simulink model "IEEE30_case"  (R2024b)
settings: Solver=FixedStepAuto  StartTime=0  StopTime=5  FixedStep=1e-7  RelTol=1e-3
values from neighbouring files (symbols this model uses):
  GFL_DFIG_7_C_bus = 0.08    [IEEE30_case_parameters.m]
  GFL_DFIG_7_D_mutual = 2.500000e+3    (= 2500)    [IEEE30_case_parameters.m]
  GFL_DFIG_7_f0 = 60    [IEEE30_case_parameters.m]
  GFL_DFIG_7_gPLLi = 3200    [IEEE30_case_parameters.m]
  GFL_DFIG_7_gPLLp = 650    [IEEE30_case_parameters.m]
  GFL_DFIG_7_H_WT = 0.4    [IEEE30_case_parameters.m]
  GFL_DFIG_7_Hg = 0.8    [IEEE30_case_parameters.m]
  GFL_DFIG_7_Igq_ref = 0    [IEEE30_case_parameters.m]
  GFL_DFIG_7_Ird_ref = 704.45696    [IEEE30_case_parameters.m]
  GFL_DFIG_7_KI_V = -300000    [IEEE30_case_parameters.m]
  GFL_DFIG_7_KP_V = -1000    [IEEE30_case_parameters.m]
  GFL_DFIG_7_Ksh = 1.254300e+4    (= 12543)    [IEEE30_case_parameters.m]
  GFL_DFIG_7_Lg = 0.000483    [IEEE30_case_parameters.m]
  GFL_DFIG_7_Lm_pu = 4    [IEEE30_case_parameters.m]
  GFL_DFIG_7_N = 100    [IEEE30_case_parameters.m]
  GFL_DFIG_7_p = 2    [IEEE30_case_parameters.m]
  GFL_DFIG_7_Pitch = 0    [IEEE30_case_parameters.m]
  GFL_DFIG_7_R = 44    [IEEE30_case_parameters.m]
  GFL_DFIG_7_Rg = 2.000000e-5    (= 2e-05)    [IEEE30_case_parameters.m]
  GFL_DFIG_7_rho = 1.225    [IEEE30_case_parameters.m]
  GFL_DFIG_7_rPLLi = 4500    [IEEE30_case_parameters.m]
  GFL_DFIG_7_rPLLp = 620    [IEEE30_case_parameters.m]
  GFL_DFIG_7_Rs_pu = 0.011    [IEEE30_case_parameters.m]
  GFL_DFIG_7_Sbase = 2.000000e+6    (= 2000000)    [IEEE30_case_parameters.m]
  GFL_DFIG_7_ugq_ref = 0    [IEEE30_case_parameters.m]
  GFL_DFIG_7_usd_ref = 0    [IEEE30_case_parameters.m]
  GFL_DFIG_7_Vbase = 690    [IEEE30_case_parameters.m]
  GFL_DFIG_7_Vdc_ref = 1200    [IEEE30_case_parameters.m]
  GFL_DFIG_7_wind = 12    [IEEE30_case_parameters.m]
  GFL_DFIG_7_wm_ref = 518.184209    [IEEE30_case_parameters.m]
  SG_D_13_D = 0.01056    [IEEE30_case_parameters.m]
  SG_D_13_EnableSaturation = 0    [IEEE30_case_parameters.m]
  SG_D_13_f0 = 60    [IEEE30_case_parameters.m]
  SG_D_13_H = 7.5    [IEEE30_case_parameters.m]
  SG_D_13_K_A = 20    [IEEE30_case_parameters.m]
  SG_D_13_K_E = 1.000000e+1    (= 10)    [IEEE30_case_parameters.m]
  SG_D_13_K_F = 2.363    [IEEE30_case_parameters.m]
  SG_D_13_K_s = 0.5    [IEEE30_case_parameters.m]
  SG_D_13_R_a = 0.001088    [IEEE30_case_parameters.m]
  SG_D_13_S_A = 1    [IEEE30_case_parameters.m]
  SG_D_13_S_B = 0.103    [IEEE30_case_parameters.m]
  SG_D_13_S_N = 10.659857    [IEEE30_case_parameters.m]
  SG_D_13_SpeedPara = 200    [IEEE30_case_parameters.m]
  SG_D_13_T_0 = 0.370163    [IEEE30_case_parameters.m]
  SG_D_13_T_1 = 0.3    [IEEE30_case_parameters.m]
  SG_D_13_T_2 = 0.05    [IEEE30_case_parameters.m]
  SG_D_13_T_3 = 0.02    [IEEE30_case_parameters.m]
  SG_D_13_T_4 = 0.005    [IEEE30_case_parameters.m]
  SG_D_13_T_A = 0.02    [IEEE30_case_parameters.m]
  SG_D_13_T_dd = 8.000000e+0    (= 8)    [IEEE30_case_parameters.m]
  SG_D_13_T_ddd = 0.04    [IEEE30_case_parameters.m]
  SG_D_13_T_E = 0.314    [IEEE30_case_parameters.m]
  SG_D_13_T_F = 0.35    [IEEE30_case_parameters.m]
  SG_D_13_T_qd = 0.8    [IEEE30_case_parameters.m]
  SG_D_13_T_qdd = 0.02    [IEEE30_case_parameters.m]
  SG_D_13_T_speed = 0.1    [IEEE30_case_parameters.m]
  SG_D_13_T_w = 0.5    [IEEE30_case_parameters.m]
  SG_D_13_V_ref = 1.696619    [IEEE30_case_parameters.m]
  SG_D_13_w_ref = 376.991118    [IEEE30_case_parameters.m]
  SG_D_13_x_d = 1.9    [IEEE30_case_parameters.m]
  SG_D_13_x_dd = 0.302    [IEEE30_case_parameters.m]
  SG_D_13_x_ddd = 0.204    [IEEE30_case_parameters.m]
  SG_D_13_x_l = 0.05    [IEEE30_case_parameters.m]
  SG_D_13_x_q = 1.3    [IEEE30_case_parameters.m]
  SG_D_13_x_qd = 0.5    [IEEE30_case_parameters.m]
  SG_D_13_x_qdd = 0.3    [IEEE30_case_parameters.m]
  SG_D_1_D = 0.01056    [IEEE30_case_parameters.m]
  SG_D_1_EnableSaturation = 0    [IEEE30_case_parameters.m]
  SG_D_1_f0 = 60    [IEEE30_case_parameters.m]
  SG_D_1_H = 7.5    [IEEE30_case_parameters.m]
  SG_D_1_K_A = 20    [IEEE30_case_parameters.m]
  SG_D_1_K_E = 1.000000e+1    (= 10)    [IEEE30_case_parameters.m]
  SG_D_1_K_F = 2.363    [IEEE30_case_parameters.m]
  SG_D_1_K_s = 0.5    [IEEE30_case_parameters.m]
  SG_D_1_R_a = 0.001088    [IEEE30_case_parameters.m]
  SG_D_1_S_A = 1    [IEEE30_case_parameters.m]
  SG_D_1_S_B = 0.103    [IEEE30_case_parameters.m]
  SG_D_1_S_N = 10.659857    [IEEE30_case_parameters.m]
  SG_D_1_SpeedPara = 200    [IEEE30_case_parameters.m]
  SG_D_1_T_0 = 0.259812    [IEEE30_case_parameters.m]
  SG_D_1_T_1 = 0.3    [IEEE30_case_parameters.m]
  SG_D_1_T_2 = 0.05    [IEEE30_case_parameters.m]
  SG_D_1_T_3 = 0.02    [IEEE30_case_parameters.m]
  SG_D_1_T_4 = 0.005    [IEEE30_case_parameters.m]
  SG_D_1_T_A = 0.02    [IEEE30_case_parameters.m]
  SG_D_1_T_dd = 8.000000e+0    (= 8)    [IEEE30_case_parameters.m]
  SG_D_1_T_ddd = 0.04    [IEEE30_case_parameters.m]
  SG_D_1_T_E = 0.314    [IEEE30_case_parameters.m]
  SG_D_1_T_F = 0.35    [IEEE30_case_parameters.m]
  SG_D_1_T_qd = 0.8    [IEEE30_case_parameters.m]
  SG_D_1_T_qdd = 0.02    [IEEE30_case_parameters.m]
  SG_D_1_T_speed = 0.1    [IEEE30_case_parameters.m]
  SG_D_1_T_w = 0.5    [IEEE30_case_parameters.m]
  SG_D_1_V_ref = 1.544107    [IEEE30_case_parameters.m]
  SG_D_1_w_ref = 376.991118    [IEEE30_case_parameters.m]
  SG_D_1_x_d = 1.9    [IEEE30_case_parameters.m]
  SG_D_1_x_dd = 0.302    [IEEE30_case_parameters.m]
  SG_D_1_x_ddd = 0.204    [IEEE30_case_parameters.m]
  SG_D_1_x_l = 0.05    [IEEE30_case_parameters.m]
  SG_D_1_x_q = 1.3    [IEEE30_case_parameters.m]
  SG_D_1_x_qd = 0.5    [IEEE30_case_parameters.m]
  SG_D_1_x_qdd = 0.3    [IEEE30_case_parameters.m]
  SG_D_22_D = 0.01056    [IEEE30_case_parameters.m]
  SG_D_22_EnableSaturation = 0    [IEEE30_case_parameters.m]
  SG_D_22_f0 = 60    [IEEE30_case_parameters.m]
  SG_D_22_H = 7.5    [IEEE30_case_parameters.m]
  SG_D_22_K_A = 20    [IEEE30_case_parameters.m]
  SG_D_22_K_E = 1.000000e+1    (= 10)    [IEEE30_case_parameters.m]
  SG_D_22_K_F = 2.363    [IEEE30_case_parameters.m]
  SG_D_22_K_s = 0.5    [IEEE30_case_parameters.m]
  SG_D_22_R_a = 0.001088    [IEEE30_case_parameters.m]
  SG_D_22_S_A = 1    [IEEE30_case_parameters.m]
  SG_D_22_S_B = 0.103    [IEEE30_case_parameters.m]
  SG_D_22_S_N = 10.659857    [IEEE30_case_parameters.m]
  SG_D_22_SpeedPara = 200    [IEEE30_case_parameters.m]
  SG_D_22_T_0 = 0.216121    [IEEE30_case_parameters.m]
  SG_D_22_T_1 = 0.3    [IEEE30_case_parameters.m]
  SG_D_22_T_2 = 0.05    [IEEE30_case_parameters.m]
  SG_D_22_T_3 = 0.02    [IEEE30_case_parameters.m]
  SG_D_22_T_4 = 0.005    [IEEE30_case_parameters.m]
  ... (+126 more)
(part 13 of 27)

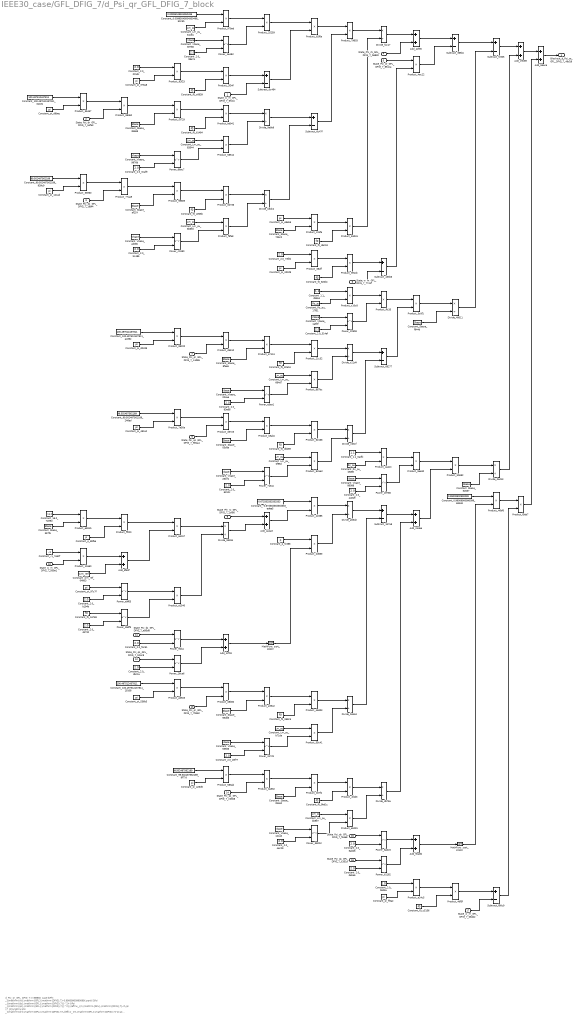
== system IEEE30_case/GFL_DFIG_7/d_Psi_qr_GFL_DFIG_7_block ==
  note: d_Psi_qr_GFL_DFIG_7 in IEEE30_case
      | $\Phi _{\mathrm{rb},\mathrm{GFL},\mathrm{DFIG},7}-0.99009900990099\,\sqrt{{\Psi _{\mathrm{ds},\mathrm{GFL},\mathrm{DFIG},7}}^2+{\Psi _{\mathrm{qs},\mathrm{GFL},\mathrm{DFIG},7}}^2}\,\left(w_{m,\mathrm{GFL},\mathrm{DFIG},7}-2\,\pi \,f_{0}\right)+\Psi _{\mathrm{dr},\mathrm{GFL},\mathrm{DFIG},7}\,\left(w_{m,\mathrm{GFL},\mathrm{DFIG},7}-2\,\pi \,f_{0}\right)-\frac{1.1\,\mathrm{Rs}_{\mathrm{pu}}\,{\mathrm{Vbase}}^2\,\left(\frac{100.497512437811\,\pi \,\Psi _{\mathrm{qr},\mathrm{GFL},\mathrm{DFIG},7}\,\mathrm{Sbase}\,f_{0}}{\mathrm{Lm}_{\mathrm{pu}}\,{\mathrm{Vbase}}^2}-\frac{99.502487562189\,\pi \,\Psi _{\mathrm{qs},\mathrm{GFL},\mathrm{DFIG},7}\,\mathrm{Sbase}\,f_{0}}{\mathrm{Lm}_{\mathrm{pu}}\,{\mathrm{Vbase}}^2}\right)}{\mathrm{Sbase}}-\frac{1.1\,\mathrm{Rs}_{\mathrm{pu}}\,{\mathrm{Vbase}}^2\,\left(\frac{0.673333333333333\,\Phi _{\mathrm{rc},\mathrm{GFL},\mathrm{DFIG},7}-\frac{10.773333333333328\,\mathrm{Sbase}\,p\,\left(w_{m,\mathrm{GFL},\mathrm{DFIG},7}-\mathrm{wm}_{\mathrm{ref}}\right)}{{f_{0}}^2\,\pi ^2}}{p\,\sqrt{{\Psi _{\mathrm{ds},\mathrm{GFL},\mathrm{DFIG},7}}^2+{\Psi _{\mathrm{qs},\mathrm{GFL},\mathrm{DFIG},7}}^2}}+\frac{100.497512437811\,\pi \,\Psi _{\mathrm{qr},\mathrm{GFL},\mathrm{DFIG},7}\,\mathrm{Sbase}\,f_{0}}{\mathrm{Lm}_{\mathrm{pu}}\,{\mathrm{Vbase}}^2}-\frac{99.502487562189\,\pi \,\Psi _{\mathrm{qs},\mathrm{GFL},\mathrm{DFIG},7}\,\mathrm{Sbase}\,f_{0}}{\mathrm{Lm}_{\mathrm{pu}}\,{\mathrm{Vbase}}^2}\right)}{\mathrm{Sbase}}-\frac{0.00995049504950496\,\mathrm{Lm}_{\mathrm{pu}}\,{\mathrm{Vbase}}^2\,\left(\frac{100.497512437811\,\pi \,\Psi _{\mathrm{dr},\mathrm{GFL},\mathrm{DFIG},7}\,\mathrm{Sbase}\,f_{0}}{\mathrm{Lm}_{\mathrm{pu}}\,{\mathrm{Vbase}}^2}-\frac{99.502487562189\,\pi \,\Psi _{\mathrm{ds},\mathrm{GFL},\mathrm{DFIG},7}\,\mathrm{Sbase}\,f_{0}}{\mathrm{Lm}_{\mathrm{pu}}\,{\mathrm{Vbase}}^2}\right)\,\left(w_{m,\mathrm{GFL},\mathrm{DFIG},7}-2\,\pi \,f_{0}\right)}{\mathrm{Sbase}\,f_{0}\,\pi }$
      | Automatically generated on 2025-11-01 18:33:02 .
  State_w_m_GFL_DFIG_7_5fc1b : Inport
  State_Psi_dr_GFL_DFIG_7_54fa3 : Inport  Port=2
  State_Psi_ds_GFL_DFIG_7_18bf4 : Inport  Port=3
  State_Phi_rb_GFL_DFIG_7_b6830 : Inport  Port=4
  State_Psi_dr_GFL_DFIG_7_851ca : Inport  Port=5
  State_w_m_GFL_DFIG_7_7741f : Inport  Port=6
  State_Psi_qr_GFL_DFIG_7_c4d86 : Inport  Port=7
  State_Psi_qs_GFL_DFIG_7_981a4 : Inport  Port=8
  State_Phi_rc_GFL_DFIG_7_1cf80 : Inport  Port=9
  State_w_m_GFL_DFIG_7_509a1 : Inport  Port=10
  State_Psi_ds_GFL_DFIG_7_e95d8 : Inport  Port=11
  State_Psi_qs_GFL_DFIG_7_b24c8 : Inport  Port=12
  State_Psi_qr_GFL_DFIG_7_7bb62 : Inport  Port=13
  State_Psi_qs_GFL_DFIG_7_c0308 : Inport  Port=14
  State_Psi_ds_GFL_DFIG_7_fa3e8 : Inport  Port=15
  State_Psi_qs_GFL_DFIG_7_c351a : Inport  Port=16
  State_w_m_GFL_DFIG_7_084b2 : Inport  Port=17
  Add_1cf03 : Sum
  Add_24dee : Sum
  Add_42f35 : Sum
  Add_4a1a3 : Sum
  Add_55ace : Sum
  Add_8fe3f : Sum
  Add_9ca6b : Sum
  Add_c9c89 : Sum
  Constant_-0.673333333333333_edee5 : Constant  Value=-0.673333333333333
  Constant_-1_7e52f : Constant  Value=-1
  Constant_0.00995049504950496_52c5b : Constant  Value=0.00995049504950496
  Constant_0.99009900990099_a5b48 : Constant  Value=0.99009900990099
  Constant_1.1_0adfc : Constant  Value=1.1
  Constant_1.1_db8a1 : Constant  Value=1.1
  Constant_100.497512437811_19108 : Constant  Value=100.497512437811
  Constant_100.497512437811_34181 : Constant  Value=100.497512437811
  Constant_100.497512437811_a4362 : Constant  Value=100.497512437811
  Constant_16.0_72e9d : Constant  Value=16.0
  Constant_2.0_001dc : Constant  Value=2.0
  Constant_2.0_0caf9 : Constant  Value=2.0
  Constant_2.0_28f77 : Constant  Value=2.0
  Constant_2.0_314ef : Constant  Value=2.0
  Constant_2.0_44819 : Constant  Value=2.0
  Constant_2.0_4b732 : Constant  Value=2.0
  Constant_2.0_4ec29 : Constant  Value=2.0
  Constant_2.0_5abb6 : Constant  Value=2.0
  Constant_2.0_6312c : Constant  Value=2.0
  Constant_2.0_73f2b : Constant  Value=2.0
  Constant_2.0_83e68 : Constant  Value=2.0
  Constant_2.0_99e74 : Constant  Value=2.0
  Constant_2.0_b194b : Constant  Value=2.0
  Constant_2.0_b505a : Constant  Value=2.0
  Constant_2.0_bc485 : Constant  Value=2.0
  Constant_2.0_dbc1a : Constant  Value=2.0
  Constant_2.0_deba6 : Constant  Value=2.0
  Constant_2.0_f4c51 : Constant  Value=2.0
  Constant_99.502487562189_246ed : Constant  Value=99.502487562189
  Constant_99.502487562189_939c9 : Constant  Value=99.502487562189
  Constant_99.502487562189_9f77d : Constant  Value=99.502487562189
  Constant_Lm_pu_0f95d : Constant  Value=Lm_pu
  Constant_Lm_pu_664d7 : Constant  Value=Lm_pu
  Constant_Lm_pu_83544 : Constant  Value=Lm_pu
  Constant_Lm_pu_8b6ed : Constant  Value=Lm_pu
  Constant_Lm_pu_b71da : Constant  Value=Lm_pu
  Constant_Lm_pu_bb9e7 : Constant  Value=Lm_pu
  Constant_Lm_pu_e4c81 : Constant  Value=Lm_pu
  Constant_Rs_pu_17f51 : Constant  Value=Rs_pu
  Constant_Rs_pu_b58f8 : Constant  Value=Rs_pu
  Constant_Sbase_05cea : Constant  Value=Sbase
  Constant_Sbase_0ba52 : Constant  Value=Sbase
  Constant_Sbase_357fe : Constant  Value=Sbase
  Constant_Sbase_3b669 : Constant  Value=Sbase
  Constant_Sbase_52637 : Constant  Value=Sbase
  Constant_Sbase_705c0 : Constant  Value=Sbase
  Constant_Sbase_8fae6 : Constant  Value=Sbase
  Constant_Sbase_9ed05 : Constant  Value=Sbase
  Constant_Sbase_af214 : Constant  Value=Sbase
  Constant_Sbase_f944d : Constant  Value=Sbase
  Constant_Vbase_12ca0 : Constant  Value=Vbase
  Constant_Vbase_1ae0f : Constant  Value=Vbase
  Constant_Vbase_204ae : Constant  Value=Vbase
  Constant_Vbase_25b72 : Constant  Value=Vbase
  Constant_Vbase_3e766 : Constant  Value=Vbase
  Constant_Vbase_55566 : Constant  Value=Vbase
  Constant_Vbase_860d8 : Constant  Value=Vbase
  Constant_Vbase_9976d : Constant  Value=Vbase
  Constant_Vbase_ad08c : Constant  Value=Vbase
  Constant_f0_068c5 : Constant  Value=f0
  Constant_f0_16769 : Constant  Value=f0
  Constant_f0_32a04 : Constant  Value=f0
  Constant_f0_4e06b : Constant  Value=f0
  Constant_f0_820bc : Constant  Value=f0
  Constant_f0_9bd1c : Constant  Value=f0
  Constant_f0_b1484 : Constant  Value=f0
  Constant_f0_c5156 : Constant  Value=f0
  Constant_f0_c6639 : Constant  Value=f0
  Constant_f0_d6c18 : Constant  Value=f0
  Constant_f0_dbb69 : Constant  Value=f0
  Constant_p_6bf5e : Constant  Value=p
  Constant_p_fc388 : Constant  Value=p
  Constant_pi_12cad : Constant  Value=pi
  Constant_pi_2d2d9 : Constant  Value=pi
  Constant_pi_37ea8 : Constant  Value=pi
  Constant_pi_426d6 : Constant  Value=pi
  Constant_pi_491a2 : Constant  Value=pi
  Constant_pi_536b5 : Constant  Value=pi
  Constant_pi_97c7f : Constant  Value=pi
  Constant_pi_d0c89 : Constant  Value=pi
  Constant_pi_d9bec : Constant  Value=pi
  Constant_pi_e9eb6 : Constant  Value=pi
  Constant_pi_ff3a2 : Constant  Value=pi
  Constant_wm_ref_04b03 : Constant  Value=wm_ref
  Divide_0ad13 : Product  Inputs=*/
  Divide_48011 : Product  Inputs=*/
  Divide_93334 : Product  Inputs=*/
  Divide_9abb9 : Product  Inputs=*/
  Divide_a55d2 : Product  Inputs=*/
  Divide_b34a3 : Product  Inputs=*/
  Divide_b3dc2 : Product  Inputs=*/
  Divide_c03cf : Product  Inputs=*/
  Divide_c21d4 : Product  Inputs=*/
  Divide_db75a : Product  Inputs=*/
  Divide_f4c17 : Product  Inputs=*/
  MathFunc_sqrt_20207 : Sqrt
  MathFunc_sqrt_c0122 : Sqrt
  Power_1e48d : Math  Operator=pow
  Power_225b9 : Math  Operator=pow
  Power_26ca6 : Math  Operator=pow
  Power_2e786 : Math  Operator=pow
  Power_317d1 : Math  Operator=pow
  Power_3602d : Math  Operator=pow
  Power_36df3 : Math  Operator=pow
  Power_66ac7 : Math  Operator=pow
  Power_6a0c6 : Math  Operator=pow
  Power_7161c : Math  Operator=pow
  Power_a9f63 : Math  Operator=pow
  Power_b1182 : Math  Operator=pow
  Power_c1590 : Math  Operator=pow
  Power_e3aa1 : Math  Operator=pow
  Power_ffbb4 : Math  Operator=pow
  Product_0d736 : Product
  Product_{11660,25259,35457,42385,58512,62168,79603,99220} (8 alike) : Product
  Product_21c32 : Product
  Product_2d65e : Product
  Product_2f34f : Product
  Product_384ff : Product
  Product_391dc : Product
  Product_3c0f1 : Product
  Product_3ee60 : Product
  Product_46bf0 : Product
  Product_46dd3 : Product
  Product_4a42c : Product
  Product_4ac22 : Product
  Product_4df3f : Product
  Product_4f4d3 : Product
  Product_53dc6 : Product
  Product_55c41 : Product
  Product_583ab : Product
  Product_641b7 : Product
  Product_774a9 : Product
  Product_7a50a : Product
  Product_887bc : Product
  Product_92f23 : Product
  Product_979ad : Product
  Product_98de2 : Product
  Product_9ae30 : Product
  Product_9c5ed : Product
  Product_9e8ee : Product
  Product_a0503 : Product
  Product_a24c5 : Product
  Product_a2540 : Product
  Product_a3542 : Product
  Product_a7124 : Product
  Product_b07f2 : Product
  Product_b2f6a : Product
  Product_ba532 : Product
  Product_bb592 : Product
  Product_bd941 : Product
  Product_beabc : Product
  Product_c04fe : Product
  Product_c10c8 : Product
  Product_d5510 : Product
  Product_d5723 : Product
  Product_d8b60 : Product
  Product_e5291 : Product
  Product_e831b : Product
  Product_f3729 : Product
  Product_f5eb7 : Product
  Product_f9fa8 : Product
  Product_ff020 : Product
  Product_ffc35 : Product
  Subtract_0c464 : Sum  Inputs=+-
  Subtract_1b7a8 : Sum  Inputs=+-
  Subtract_365bc : Sum  Inputs=+-
  Subtract_433b6 : Sum  Inputs=+-
  Subtract_66277 : Sum  Inputs=+-
  Subtract_6c47f : Sum  Inputs=+-
  Subtract_f80c9 : Sum  Inputs=+-
  Subtract_fc605 : Sum  Inputs=+-
  Blockout_d_Psi_qr_GFL_DFIG_7_49d19 : Outport
  wires:
  Constant_2.0_5abb6/1 -> Power_6a0c6/2
  Constant_1.1_db8a1/1 -> Product_c10c8/1
  Constant_Vbase_55566/1 -> Power_317d1/1
  State_Psi_qs_GFL_DFIG_7_b24c8/1 -> Power_26ca6/1
  Add_55ace/1 -> Blockout_d_Psi_qr_GFL_DFIG_7_49d19/1
  Constant_Lm_pu_bb9e7/1 -> Product_e5291/1
  Add_42f35/1 -> Subtract_365bc/1
  State_Psi_qr_GFL_DFIG_7_c4d86/1 -> Product_d5510/2
  Power_b1182/1 -> Add_9ca6b/2
  Power_3602d/1 -> Product_e5291/2
  Constant_Vbase_204ae/1 -> Power_e3aa1/1
  Subtract_f80c9/1 -> Product_f5eb7/2
  Product_3ee60/1 -> Product_774a9/1
  Product_42385/1 -> Divide_a55d2/1
  Product_4df3f/1 -> Subtract_f80c9/1
  Product_f5eb7/1 -> Add_55ace/2
  Constant_Lm_pu_b71da/1 -> Product_55c41/1
  Product_92f23/1 -> Product_2f34f/1
  MathFunc_sqrt_c0122/1 -> Product_46bf0/2
  Add_1cf03/1 -> MathFunc_sqrt_20207/1
  State_w_m_GFL_DFIG_7_084b2/1 -> Subtract_f80c9/2
  Divide_a55d2/1 -> Subtract_1b7a8/1
  Product_46bf0/1 -> Product_f5eb7/1
  Constant_2.0_dbc1a/1 -> Power_26ca6/2
  Product_11660/1 -> Add_8fe3f/1
  Add_24dee/1 -> Product_bb592/2
  Constant_Vbase_12ca0/1 -> Power_3602d/1
  Constant_0.99009900990099_a5b48/1 -> Product_46bf0/1
  Constant_f0_c5156/1 -> Product_4df3f/2
  Add_9ca6b/1 -> MathFunc_sqrt_c0122/1
  Constant_p_fc388/1 -> Product_2d65e/1
  Constant_pi_ff3a2/1 -> Product_a24c5/2
  Constant_Sbase_0ba52/1 -> Product_b07f2/2
  Product_a24c5/1 -> Product_4df3f/1
  Product_9ae30/1 -> Product_bb592/1
  Constant_2.0_b505a/1 -> Product_a24c5/1
  Power_317d1/1 -> Product_55c41/2
  Constant_pi_426d6/1 -> Product_583ab/2
  Divide_0ad13/1 -> Add_c9c89/2
  State_Psi_qs_GFL_DFIG_7_c351a/1 -> Power_b1182/1
  Product_ba532/1 -> Product_b07f2/1
  Constant_100.497512437811_19108/1 -> Product_a0503/1
  State_Phi_rb_GFL_DFIG_7_b6830/1 -> Add_42f35/2
  Constant_2.0_deba6/1 -> Power_b1182/2
  Constant_2.0_0caf9/1 -> Power_66ac7/2
  Constant_Vbase_1ae0f/1 -> Power_225b9/1
  State_Psi_qs_GFL_DFIG_7_c0308/1 -> Product_ba532/2
  Divide_db75a/1 -> Add_24dee/2
  Product_53dc6/1 -> Divide_f4c17/2
  Product_21c32/1 -> Divide_c21d4/1
  Constant_99.502487562189_9f77d/1 -> Product_583ab/1
  Constant_100.497512437811_34181/1 -> Product_35457/1
  Constant_f0_9bd1c/1 -> Product_4f4d3/2
  Constant_pi_d0c89/1 -> Product_99220/2
  Power_6a0c6/1 -> Add_9ca6b/1
  Product_bb592/1 -> Divide_0ad13/1
  Product_bd941/1 -> Divide_9abb9/1
  Product_583ab/1 -> Product_ba532/1
  Product_9c5ed/1 -> Divide_c03cf/2
  Product_98de2/1 -> Product_f3729/1
  State_Psi_ds_GFL_DFIG_7_fa3e8/1 -> Power_6a0c6/1
  Product_b07f2/1 -> Product_4f4d3/1
  Add_8fe3f/1 -> Product_641b7/2
  Constant_f0_d6c18/1 -> Product_53dc6/2
  Constant_f0_068c5/1 -> Product_46dd3/2
  Constant_Sbase_52637/1 -> Divide_0ad13/2
  Add_c9c89/1 -> Add_55ace/1
  Product_46dd3/1 -> Divide_b34a3/1
  Constant_2.0_314ef/1 -> Power_225b9/2
  Product_e5291/1 -> Divide_db75a/2
  Constant_2.0_4ec29/1 -> Power_3602d/2
  Product_4f4d3/1 -> Divide_db75a/1
  Product_4ac22/1 -> Subtract_365bc/2
  Constant_pi_536b5/1 -> Product_a0503/2
  Subtract_1b7a8/1 -> Add_24dee/1
  Constant_pi_2d2d9/1 -> Product_384ff/2
  Product_391dc/1 -> Subtract_433b6/1
  Constant_f0_820bc/1 -> Product_391dc/2
  Divide_b34a3/1 -> Subtract_1b7a8/2
  Product_55c41/1 -> Divide_b34a3/2
  Constant_2.0_28f77/1 -> Power_317d1/2
  Product_a3542/1 -> Product_46dd3/1
  Constant_2.0_f4c51/1 -> Power_ffbb4/2
  Constant_Sbase_9ed05/1 -> Product_a3542/2
  Power_ffbb4/1 -> Add_1cf03/1
  Product_d8b60/1 -> Product_a3542/1
  State_Psi_qr_GFL_DFIG_7_7bb62/1 -> Product_d8b60/2
  Product_a0503/1 -> Product_d8b60/1
  Product_2d65e/1 -> Divide_a55d2/2
  MathFunc_sqrt_20207/1 -> Product_2d65e/2
  Constant_Vbase_3e766/1 -> Power_1e48d/1
  Power_26ca6/1 -> Add_1cf03/2
  Product_f9fa8/1 -> Divide_b3dc2/2
  State_Psi_ds_GFL_DFIG_7_e95d8/1 -> Power_ffbb4/1
  Constant_pi_e9eb6/1 -> Product_c04fe/1
  Constant_2.0_44819/1 -> Power_2e786/2
  Add_4a1a3/1 -> Product_42385/2
  Power_7161c/1 -> Product_9c5ed/2
  Divide_93334/1 -> Add_4a1a3/2
  Product_a2540/1 -> Divide_93334/2
  Constant_Sbase_05cea/1 -> Product_beabc/2
  Subtract_fc605/1 -> Add_c9c89/1
  Power_36df3/1 -> Product_a2540/2
  Constant_2.0_4b732/1 -> Power_36df3/2
  Constant_p_6bf5e/1 -> Product_ff020/2
  Constant_f0_16769/1 -> Power_36df3/1
  Power_a9f63/1 -> Product_a2540/1
  Constant_2.0_b194b/1 -> Power_a9f63/2
  Constant_Lm_pu_0f95d/1 -> Product_9c5ed/1
  Power_2e786/1 -> Product_9ae30/2
  Constant_pi_97c7f/1 -> Power_a9f63/1
  Product_641b7/1 -> Divide_93334/1
  Constant_2.0_6312c/1 -> Power_7161c/2
  Constant_wm_ref_04b03/1 -> Add_8fe3f/2
  State_w_m_GFL_DFIG_7_509a1/1 -> Product_11660/2
  Constant_-1_7e52f/1 -> Product_11660/1
  Product_ff020/1 -> Product_641b7/1
  Product_e831b/1 -> Product_ff020/1
  Product_58512/1 -> Divide_9abb9/2
  Constant_Sbase_357fe/1 -> Product_e831b/2
  Constant_16.0_72e9d/1 -> Product_e831b/1
  State_Phi_rc_GFL_DFIG_7_1cf80/1 -> Add_4a1a3/1
  Constant_-0.673333333333333_edee5/1 -> Product_42385/1
  Constant_Vbase_860d8/1 -> Power_2e786/1
  Product_4a42c/1 -> Product_9ae30/1
  Product_2f34f/1 -> Subtract_0c464/1
  Constant_Rs_pu_b58f8/1 -> Product_4a42c/2
  Constant_1.1_0adfc/1 -> Product_4a42c/1
  Divide_48011/1 -> Subtract_fc605/2
  Subtract_6c47f/1 -> Product_79603/2
  Constant_Sbase_f944d/1 -> Divide_48011/2
  Product_3c0f1/1 -> Divide_48011/1
  Subtract_66277/1 -> Product_3c0f1/2
  Constant_Lm_pu_8b6ed/1 -> Product_f9fa8/1
  Product_62168/1 -> Divide_c03cf/1
  Divide_c03cf/1 -> Subtract_66277/2
  Constant_Vbase_25b72/1 -> Power_7161c/1
  Constant_f0_dbb69/1 -> Product_62168/2
  Product_beabc/1 -> Product_62168/1
  Product_d5723/1 -> Product_beabc/1
  State_Psi_qs_GFL_DFIG_7_981a4/1 -> Product_d5723/2
  Product_7a50a/1 -> Product_d5723/1
  Product_f3729/1 -> Product_bd941/1
  Constant_pi_491a2/1 -> Product_7a50a/2
  Constant_99.502487562189_246ed/1 -> Product_7a50a/1
  Divide_c21d4/1 -> Subtract_66277/1
  Product_887bc/1 -> Divide_c21d4/2
  Power_e3aa1/1 -> Product_887bc/2
  Constant_2.0_83e68/1 -> Power_e3aa1/2
  Constant_Lm_pu_664d7/1 -> Product_887bc/1
  Constant_f0_32a04/1 -> Product_21c32/2
  Product_a7124/1 -> Product_21c32/1
  Product_d5510/1 -> Product_a7124/1
  Constant_Sbase_8fae6/1 -> Product_a7124/2
  Product_99220/1 -> Product_d5510/1
  Subtract_433b6/1 -> Product_4ac22/2
  Constant_f0_c6639/1 -> Product_2f34f/2
  Constant_100.497512437811_a4362/1 -> Product_99220/1
  Product_ffc35/1 -> Product_3c0f1/1
  Power_225b9/1 -> Product_ffc35/2
  Constant_2.0_bc485/1 -> Power_c1590/2
  Product_c10c8/1 -> Product_ffc35/1
  Constant_Rs_pu_17f51/1 -> Product_c10c8/2
  Subtract_365bc/1 -> Subtract_fc605/1
  State_w_m_GFL_DFIG_7_7741f/1 -> Subtract_433b6/2
  State_Psi_ds_GFL_DFIG_7_18bf4/1 -> Product_774a9/2
  Product_384ff/1 -> Product_391dc/1
  Constant_2.0_73f2b/1 -> Product_384ff/1
  State_Psi_dr_GFL_DFIG_7_851ca/1 -> Product_4ac22/1
  Divide_f4c17/1 -> Add_42f35/1
  Product_c04fe/1 -> Product_53dc6/1
  Constant_Sbase_705c0/1 -> Product_c04fe/2
  Product_79603/1 -> Divide_f4c17/1
  Divide_b3dc2/1 -> Subtract_6c47f/2
  Power_1e48d/1 -> Product_25259/2
  Power_c1590/1 -> Product_f9fa8/2
  Constant_Vbase_ad08c/1 -> Power_c1590/1
  Product_0d736/1 -> Divide_b3dc2/1
  Constant_f0_4e06b/1 -> Product_0d736/2
  Product_9e8ee/1 -> Product_0d736/1
  Constant_Sbase_af214/1 -> Product_9e8ee/2
  Product_774a9/1 -> Product_9e8ee/1
  Constant_pi_12cad/1 -> Product_3ee60/2
  Constant_99.502487562189_939c9/1 -> Product_3ee60/1
  Divide_9abb9/1 -> Subtract_6c47f/1
  Power_66ac7/1 -> Product_58512/2
  Constant_Vbase_9976d/1 -> Power_66ac7/1
  Constant_Lm_pu_83544/1 -> Product_58512/1
  Constant_f0_b1484/1 -> Product_bd941/2
  Constant_Sbase_3b669/1 -> Product_f3729/2
  State_Psi_dr_GFL_DFIG_7_54fa3/1 -> Product_98de2/2
  Product_35457/1 -> Product_98de2/1
  Constant_pi_d9bec/1 -> Product_35457/2
  Product_b2f6a/1 -> Product_79603/1
  Subtract_0c464/1 -> Product_b2f6a/2
  State_w_m_GFL_DFIG_7_5fc1b/1 -> Subtract_0c464/2
  Constant_pi_37ea8/1 -> Product_92f23/2
  Constant_2.0_001dc/1 -> Product_92f23/1
  Product_25259/1 -> Product_b2f6a/1
  Constant_2.0_99e74/1 -> Power_1e48d/2
  Product_979ad/1 -> Product_25259/1
  Constant_Lm_pu_e4c81/1 -> Product_979ad/2
  Constant_0.00995049504950496_52c5b/1 -> Product_979ad/1

== system IEEE30_case/GFL_DFIG_7/d_Psi_qs_GFL_DFIG_7_block ==
  note: d_Psi_qs_GFL_DFIG_7 in IEEE30_case
      | $\frac{\mathrm{Rs}_{\mathrm{pu}}\,{\mathrm{Vbase}}^2\,\left(\frac{99.502487562189\,\pi \,\Psi _{\mathrm{qr},\mathrm{GFL},\mathrm{DFIG},7}\,\mathrm{Sbase}\,f_{0}}{\mathrm{Lm}_{\mathrm{pu}}\,{\mathrm{Vbase}}^2}-\frac{100.497512437811\,\pi \,\Psi _{\mathrm{qs},\mathrm{GFL},\mathrm{DFIG},7}\,\mathrm{Sbase}\,f_{0}}{\mathrm{Lm}_{\mathrm{pu}}\,{\mathrm{Vbase}}^2}\right)}{\mathrm{Sbase}}-2\,\pi \,\Psi _{\mathrm{ds},\mathrm{GFL},\mathrm{DFIG},7}\,f_{0}-\mathrm{Vbase}\,\left(v_{q,\mathrm{GFL},\mathrm{DFIG},7}\,\cos\left(\theta _{\mathrm{pllr},\mathrm{GFL},\mathrm{DFIG},7}\right)+v_{d,\mathrm{GFL},\mathrm{DFIG},7}\,\sin\left(\theta _{\mathrm{pllr},\mathrm{GFL},\mathrm{DFIG},7}\right)\right)$
      | Automatically generated on 2025-11-01 18:32:35 .
  State_Psi_ds_GFL_DFIG_7_90de9 : Inport
  State_Psi_qr_GFL_DFIG_7_e0b4f : Inport  Port=2
  State_Psi_qs_GFL_DFIG_7_b8433 : Inport  Port=3
  Input_v_d_GFL_DFIG_7_b1351 : Inport  Port=4
  State_theta_pllr_GFL_DFIG_7_5db89 : Inport  Port=5
  Input_v_q_GFL_DFIG_7_1b265 : Inport  Port=6
  State_theta_pllr_GFL_DFIG_7_ab88b : Inport  Port=7
  Add_05679 : Sum
  Add_d712b : Sum
  Constant_-1_14e2d : Constant  Value=-1
  Constant_-2.0_05158 : Constant  Value=-2.0
  Constant_-99.502487562189_0af13 : Constant  Value=-99.502487562189
  Constant_100.497512437811_b4471 : Constant  Value=100.497512437811
  Constant_2.0_05449 : Constant  Value=2.0
  Constant_2.0_29645 : Constant  Value=2.0
  Constant_2.0_2f381 : Constant  Value=2.0
  Constant_Lm_pu_31d4a : Constant  Value=Lm_pu
  Constant_Lm_pu_97a11 : Constant  Value=Lm_pu
  Constant_Rs_pu_415ee : Constant  Value=Rs_pu
  Constant_Sbase_92d1d : Constant  Value=Sbase
  Constant_Sbase_9cdbc : Constant  Value=Sbase
  Constant_Sbase_c8db8 : Constant  Value=Sbase
  Constant_Vbase_72de1 : Constant  Value=Vbase
  Constant_Vbase_7e994 : Constant  Value=Vbase
  Constant_Vbase_8fefb : Constant  Value=Vbase
  Constant_Vbase_9231f : Constant  Value=Vbase
  Constant_f0_4d31c : Constant  Value=f0
  Constant_f0_be9d9 : Constant  Value=f0
  Constant_f0_e5f2c : Constant  Value=f0
  Constant_pi_34fb3 : Constant  Value=pi
  Constant_pi_6d70d : Constant  Value=pi
  Constant_pi_ac4ca : Constant  Value=pi
  Divide_00334 : Product  Inputs=*/
  Divide_87c86 : Product  Inputs=*/
  Divide_d6566 : Product  Inputs=*/
  MathFunc_cos_a232e : Trigonometry  Operator=cos
  MathFunc_sin_5425e : Trigonometry
  Power_2ce9c : Math  Operator=pow
  Power_417a6 : Math  Operator=pow
  Power_b6549 : Math  Operator=pow
  Product_00a2d : Product
  Product_040c7 : Product
  Product_040d0 : Product
  Product_1edd5 : Product
  Product_449d0 : Product
  Product_463ea : Product
  Product_47f6c : Product
  Product_77bf5 : Product
  Product_8f966 : Product
  Product_9c47e : Product
  Product_a9de4 : Product
  Product_b44a4 : Product
  Product_cd38c : Product
  Product_cdcd9 : Product
  Product_d8018 : Product
  Product_de1a2 : Product
  Product_f0c00 : Product
  Product_f5811 : Product
  Product_fe625 : Product
  Subtract_2593a : Sum  Inputs=+-
  Subtract_39252 : Sum  Inputs=+-
  Blockout_d_Psi_qs_GFL_DFIG_7_2d6b6 : Outport
  wires:
  Constant_pi_34fb3/1 -> Product_d8018/2
  State_Psi_ds_GFL_DFIG_7_90de9/1 -> Product_9c47e/2
  Product_00a2d/1 -> Product_cdcd9/1
  Constant_-99.502487562189_0af13/1 -> Product_d8018/1
  Power_2ce9c/1 -> Product_449d0/2
  Product_d8018/1 -> Product_a9de4/1
  Constant_100.497512437811_b4471/1 -> Product_fe625/1
  Constant_Rs_pu_415ee/1 -> Product_de1a2/1
  Constant_pi_ac4ca/1 -> Product_fe625/2
  State_Psi_qr_GFL_DFIG_7_e0b4f/1 -> Product_a9de4/2
  State_Psi_qs_GFL_DFIG_7_b8433/1 -> Product_f0c00/2
  Divide_87c86/1 -> Subtract_2593a/2
  Product_8f966/1 -> Product_9c47e/1
  Product_fe625/1 -> Product_f0c00/1
  Add_05679/1 -> Blockout_d_Psi_qs_GFL_DFIG_7_2d6b6/1
  MathFunc_cos_a232e/1 -> Product_77bf5/2
  Constant_Lm_pu_31d4a/1 -> Product_449d0/1
  Product_a9de4/1 -> Product_040d0/1
  Constant_Vbase_7e994/1 -> Power_417a6/1
  Constant_Sbase_c8db8/1 -> Product_040d0/2
  Power_417a6/1 -> Product_de1a2/2
  Constant_Vbase_72de1/1 -> Power_2ce9c/1
  Product_47f6c/1 -> Divide_00334/1
  Constant_2.0_05449/1 -> Power_2ce9c/2
  Product_f0c00/1 -> Product_00a2d/1
  Product_77bf5/1 -> Subtract_39252/2
  Constant_Sbase_92d1d/1 -> Product_00a2d/2
  Constant_Vbase_9231f/1 -> Power_b6549/1
  Constant_2.0_29645/1 -> Power_b6549/2
  Constant_f0_e5f2c/1 -> Product_cdcd9/2
  Product_040d0/1 -> Product_47f6c/1
  Constant_f0_be9d9/1 -> Product_47f6c/2
  Product_cd38c/1 -> Subtract_2593a/1
  Constant_Lm_pu_97a11/1 -> Product_463ea/1
  Product_9c47e/1 -> Product_cd38c/1
  Power_b6549/1 -> Product_463ea/2
  Constant_2.0_2f381/1 -> Power_417a6/2
  Product_449d0/1 -> Divide_00334/2
  Constant_Sbase_9cdbc/1 -> Divide_87c86/2
  Product_cdcd9/1 -> Divide_d6566/1
  Product_463ea/1 -> Divide_d6566/2
  Product_f5811/1 -> Subtract_39252/1
  Constant_-2.0_05158/1 -> Product_8f966/1
  Input_v_q_GFL_DFIG_7_1b265/1 -> Product_77bf5/1
  Constant_pi_6d70d/1 -> Product_8f966/2
  Product_b44a4/1 -> Add_05679/2
  Divide_00334/1 -> Add_d712b/1
  Divide_d6566/1 -> Add_d712b/2
  Constant_-1_14e2d/1 -> Product_040c7/1
  Input_v_d_GFL_DFIG_7_b1351/1 -> Product_040c7/2
  State_theta_pllr_GFL_DFIG_7_5db89/1 -> MathFunc_sin_5425e/1
  State_theta_pllr_GFL_DFIG_7_ab88b/1 -> MathFunc_cos_a232e/1
  Subtract_39252/1 -> Product_b44a4/2
  Product_de1a2/1 -> Product_1edd5/1
  Subtract_2593a/1 -> Add_05679/1
  Add_d712b/1 -> Product_1edd5/2
  Product_1edd5/1 -> Divide_87c86/1
  Product_040c7/1 -> Product_f5811/1
  MathFunc_sin_5425e/1 -> Product_f5811/2
  Constant_f0_4d31c/1 -> Product_cd38c/2
  Constant_Vbase_8fefb/1 -> Product_b44a4/1

== system IEEE30_case/GFL_DFIG_7/d_Turbine_w_GFL_DFIG_7_block ==
  note: d_Turbine_w_GFL_DFIG_7 in IEEE30_case
      | $-\frac{\mathrm{Ksh}\,\mathrm{shaft}_{w,\mathrm{GFL},\mathrm{DFIG},7}+D_{\mathrm{mutual}}\,\left(\mathrm{Turbine}_{w,\mathrm{GFL},\mathrm{DFIG},7}-\frac{w_{m,\mathrm{GFL},\mathrm{DFIG},7}}{p}\right)+\frac{0.473147934926167\,\pi \,R^2\,\rho \,{\mathrm{wind}}^3\,{\mathrm{e}}^{-\frac{18.4\,N\,\mathrm{wind}}{R\,\mathrm{Turbine}_{w,\mathrm{GFL},\mathrm{DFIG},7}}}\,\left(\frac{110.23\,N\,\mathrm{wind}}{R\,\mathrm{Turbine}_{w,\mathrm{GFL},\mathrm{DFIG},7}}-9.30531\right)}{\mathrm{Turbine}_{w,\mathrm{GFL},\mathrm{DFIG},7}}}{2\,H_{\mathrm{WT}}}$
      | Automatically generated on 2025-11-01 18:33:07 .
  State_Turbine_w_GFL_DFIG_7_f59a7 : Inport
  State_w_m_GFL_DFIG_7_7a0a3 : Inport  Port=2
  State_shaft_w_GFL_DFIG_7_53793 : Inport  Port=3
  State_Turbine_w_GFL_DFIG_7_01506 : Inport  Port=4
  State_Turbine_w_GFL_DFIG_7_921a6 : Inport  Port=5
  State_Turbine_w_GFL_DFIG_7_deaae : Inport  Port=6
  Constant_-18.4_c388e : Constant  Value=-18.4
  Constant_-1_311e2 : Constant  Value=-1
  Constant_0.473147934926167_63cbc : Constant  Value=0.473147934926167
  Constant_110.23_73c1a : Constant  Value=110.23
  Constant_2.0_3682f : Constant  Value=2.0
  Constant_2.0_40f7a : Constant  Value=2.0
  Constant_3.0_56494 : Constant  Value=3.0
  Constant_9.30531_a1c95 : Constant  Value=9.30531
  Constant_D_mutual_69490 : Constant  Value=D_mutual
  Constant_H_WT_86001 : Constant  Value=H_WT
  Constant_Ksh_a6d2d : Constant  Value=Ksh
  Constant_N_734ff : Constant  Value=N
  Constant_N_acf05 : Constant  Value=N
  Constant_R_0c834 : Constant  Value=R
  Constant_R_261b8 : Constant  Value=R
  Constant_R_a9239 : Constant  Value=R
  Constant_p_cfe8b : Constant  Value=p
  Constant_pi_77988 : Constant  Value=pi
  Constant_rho_b6a89 : Constant  Value=rho
  Constant_wind_4ab8e : Constant  Value=wind
  Constant_wind_a4b5c : Constant  Value=wind
  Constant_wind_e6867 : Constant  Value=wind
  Divide_014ba : Product  Inputs=*/
  Divide_3cbf6 : Product  Inputs=*/
  Divide_50046 : Product  Inputs=*/
  Divide_7177d : Product  Inputs=*/
  Divide_b724f : Product  Inputs=*/
  MathFunc_exp_6f00f : Math
  Power_42979 : Math  Operator=pow
  Power_9e24f : Math  Operator=pow
  Product_0419e : Product
  Product_0c837 : Product
  Product_136fa : Product
  Product_2c8ec : Product
  Product_4d52b : Product
  Product_55d38 : Product
  Product_6d378 : Product
  Product_6efd8 : Product
  Product_9204f : Product
  Product_a2013 : Product
  Product_a68b1 : Product
  Product_aed4e : Product
  Product_ba60c : Product
  Product_df7fa : Product
  Product_e5318 : Product
  Product_e7be5 : Product
  Subtract_0d243 : Sum  Inputs=+-
  Subtract_18963 : Sum  Inputs=+-
  Subtract_46401 : Sum  Inputs=+-
  Subtract_f1b71 : Sum  Inputs=+-
  Blockout_d_Turbine_w_GFL_DFIG_7_37f45 : Outport
  wires:
  Constant_0.473147934926167_63cbc/1 -> Product_0419e/1
  Product_0c837/1 -> Divide_014ba/2
  Constant_pi_77988/1 -> Product_0419e/2
  Product_136fa/1 -> Subtract_0d243/1
  Product_0419e/1 -> Product_e7be5/1
  Product_6efd8/1 -> Divide_50046/1
  Constant_R_261b8/1 -> Power_9e24f/1
  Power_9e24f/1 -> Product_e7be5/2
  Product_a2013/1 -> Product_136fa/1
  Constant_2.0_3682f/1 -> Power_9e24f/2
  Constant_110.23_73c1a/1 -> Product_55d38/1
  Product_9204f/1 -> Subtract_0d243/2
  Subtract_18963/1 -> Product_6d378/2
  Product_ba60c/1 -> Product_6d378/1
  Constant_R_a9239/1 -> Product_aed4e/1
  Constant_N_734ff/1 -> Product_55d38/2
  Product_55d38/1 -> Product_df7fa/1
  MathFunc_exp_6f00f/1 -> Product_6efd8/2
  Constant_wind_e6867/1 -> Product_df7fa/2
  Product_a68b1/1 -> Product_ba60c/1
  State_Turbine_w_GFL_DFIG_7_01506/1 -> Product_aed4e/2
  Constant_R_0c834/1 -> Product_0c837/1
  Constant_-18.4_c388e/1 -> Product_4d52b/1
  Constant_-1_311e2/1 -> Product_a2013/1
  Constant_N_acf05/1 -> Product_4d52b/2
  Product_e7be5/1 -> Product_a68b1/1
  Product_e5318/1 -> Divide_3cbf6/2
  Subtract_f1b71/1 -> Product_136fa/2
  Power_42979/1 -> Product_ba60c/2
  Constant_rho_b6a89/1 -> Product_a68b1/2
  Constant_p_cfe8b/1 -> Divide_7177d/2
  Constant_wind_a4b5c/1 -> Power_42979/1
  Product_6d378/1 -> Product_6efd8/1
  Constant_3.0_56494/1 -> Power_42979/2
  Product_df7fa/1 -> Divide_b724f/1
  Product_aed4e/1 -> Divide_b724f/2
  Product_4d52b/1 -> Product_2c8ec/1
  Divide_3cbf6/1 -> Blockout_d_Turbine_w_GFL_DFIG_7_37f45/1
  Constant_wind_4ab8e/1 -> Product_2c8ec/2
  Divide_b724f/1 -> Subtract_18963/1
  State_Turbine_w_GFL_DFIG_7_921a6/1 -> Product_0c837/2
  State_w_m_GFL_DFIG_7_7a0a3/1 -> Divide_7177d/1
  Constant_9.30531_a1c95/1 -> Subtract_18963/2
  Constant_D_mutual_69490/1 -> Product_a2013/2
  Product_2c8ec/1 -> Divide_014ba/1
  State_Turbine_w_GFL_DFIG_7_f59a7/1 -> Subtract_f1b71/1
  Divide_7177d/1 -> Subtract_f1b71/2
  Divide_014ba/1 -> MathFunc_exp_6f00f/1
  Constant_Ksh_a6d2d/1 -> Product_9204f/1
  Constant_2.0_40f7a/1 -> Product_e5318/1
  State_shaft_w_GFL_DFIG_7_53793/1 -> Product_9204f/2
  State_Turbine_w_GFL_DFIG_7_deaae/1 -> Divide_50046/2
  Subtract_0d243/1 -> Subtract_46401/1
  Divide_50046/1 -> Subtract_46401/2
  Constant_H_WT_86001/1 -> Product_e5318/2
  Subtract_46401/1 -> Divide_3cbf6/1
